simulink model "sampled_data_system"  (R2020a)
settings: Solver=VariableStepAuto  StartTime=0.0  StopTime=20  RelTol=1e-3
values from neighbouring files (symbols this model uses):
  B = 1 / k_m    (= 0.0517063081696)    [Teleop_parameters.m]    (also in base.mat; base_no_attrito.mat = 0; ci_siamo.mat; force_control.mat)
  Be = 5    [Teleop_parameters.m]    (also in base.mat = 0.5; base_no_attrito.mat = 0.5; ci_siamo.mat; force_control.mat = 0.5)
  Bh = 0.02    [Teleop_parameters.m]    (also in base.mat; base_no_attrito.mat; ci_siamo.mat; force_control.mat)
  D = 1    [Teleop_parameters.m]    (also in base.mat = 2; base_no_attrito.mat = 2; force_control.mat = 2; force_control_senza_attrito.mat = 2)
  Fc_h = 5    [Teleop_parameters.m]    (also in base.mat; base_no_attrito.mat; ci_siamo.mat; force_control.mat)
  J = tau_m / k_m    (= 0.0629265770424)    [Teleop_parameters.m]    (also in base.mat; base_no_attrito.mat; ci_siamo.mat; force_control.mat)
  J_r = J + J * 0.5    (= 0.0943898655636)    [Teleop_parameters.m]    (also in base.mat; base_no_attrito.mat; ci_siamo.mat = 0.0629265770424; force_control.mat)
  Jh = 0.02    [Teleop_parameters.m]    (also in base.mat; base_no_attrito.mat; ci_siamo.mat; force_control.mat)
  Kc2v_m = 2    [Teleop_parameters.m]    (also in base.mat; base_no_attrito.mat; ci_siamo.mat; force_control.mat)
  Kc2v_s = 2    [Teleop_parameters.m]    (also in base.mat; base_no_attrito.mat; ci_siamo.mat; force_control.mat)
  Kd_h = 1    [Teleop_parameters.m]    (also in base.mat; base_no_attrito.mat; ci_siamo.mat = 10; force_control.mat)
  Kd_m = 1    [Teleop_parameters.m]    (also in base.mat; base_no_attrito.mat; ci_siamo.mat = 0.005; force_control.mat)
  Kd_s = 1    [Teleop_parameters.m]    (also in base.mat; base_no_attrito.mat; ci_siamo.mat = 0.5; force_control.mat)
  Ke = 10    [Teleop_parameters.m]    (also in base.mat; base_no_attrito.mat; ci_siamo.mat; force_control.mat)
  Kp_h = 1.2    [Teleop_parameters.m]    (also in base.mat; base_no_attrito.mat; ci_siamo.mat = 10; force_control.mat)
  Kp_m = 1    [Teleop_parameters.m]    (also in base.mat; base_no_attrito.mat; ci_siamo.mat = 0.01; force_control.mat)
  Kp_s = 1    [Teleop_parameters.m]    (also in base.mat; base_no_attrito.mat; ci_siamo.mat; force_control.mat)
  Kt2c_m = 1.182    [Teleop_parameters.m]    (also in base.mat; base_no_attrito.mat; ci_siamo.mat; force_control.mat)
  Kt2c_s = 1.182    [Teleop_parameters.m]    (also in base.mat; base_no_attrito.mat; ci_siamo.mat; force_control.mat)
  Kv_fc = 0    [Teleop_parameters.m]    (also in base.mat; base_no_attrito.mat; ci_siamo.mat = 10; force_control.mat = 30)
  lArm_m = 0.1    [Teleop_parameters.m]    (also in base.mat; base_no_attrito.mat; ci_siamo.mat; force_control.mat)
  lArm_s = 0.1    [Teleop_parameters.m]    (also in base.mat; base_no_attrito.mat; ci_siamo.mat; force_control.mat)
  qe = 0.5    [Teleop_parameters.m]    (also in base.mat = 5; base_no_attrito.mat = 5; ci_siamo.mat; force_control.mat = 5)
  Ts = 0.002    [Teleop_parameters.m]    (also in base.mat; base_no_attrito.mat; ci_siamo.mat; force_control.mat)
undefined symbols (not defined in the file or in its folder): DiscIntNeverNeededParam
settings Model: Creator=gbagolin  LastModifiedBy=giova
settings SolverCC: AlgebraicLoopSolver=LineSearch

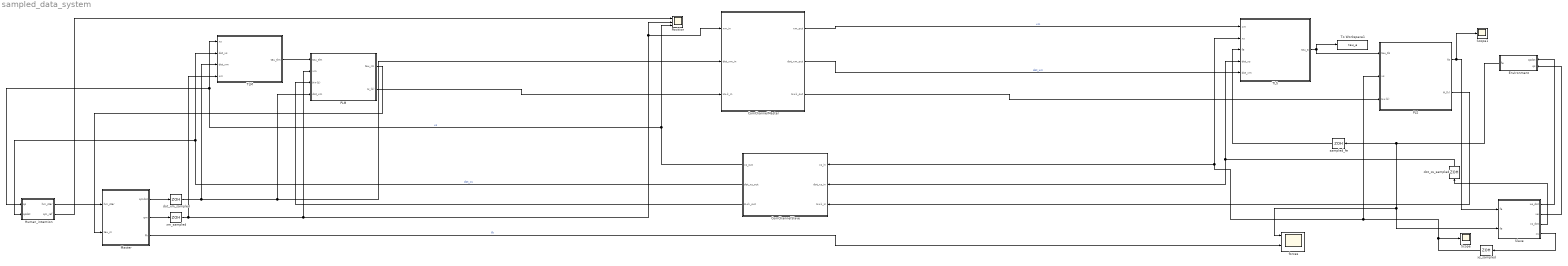
== system sampled_data_system ==
  ComChannelMaster : Subsystem
  ComChannelSlave : Subsystem
  Environment : Subsystem
  Human_intention : Subsystem
  Master : Subsystem
  PLM : Subsystem
  PLS : Subsystem
  Position : Scope  NumInputPorts=3
  Scope : Scope
  Scope1 : Scope
  Slave : Subsystem
  TLM : Subsystem
  TLS : Subsystem
  To Workspace1 : ToWorkspace  VariableName=tau_a  SaveFormat=Timeseries  SampleTime=-1
  dot_xm_sampled : ZeroOrderHold  SampleTime=Ts
  dot_xs_sampled : ZeroOrderHold  SampleTime=Ts
  forces : Scope  NumInputPorts=5
  sampled_fe : ZeroOrderHold  SampleTime=-1
  xm_sampled : ZeroOrderHold  SampleTime=Ts
  xs_sampled : ZeroOrderHold  SampleTime=Ts
  wires:
  Human_intention/1(hm_star) -> Master/1(hm_star)
  Environment/1(fe) -> Slave/2(fe), forces/1, sampled_fe/1
  Slave/3(xs_dot) -> dot_xs_sampled/1
  Slave/1(xe_dot) -> Environment/1(qsdot)
  Slave/2(xe) -> Environment/2(qs)
  Slave/4(xs) -> xs_sampled/1
  Master/2(qm) -> xm_sampled/1
  Human_intention/2(qm_ref) -> Position/1
  Master/3(fh) -> forces/4  "fh"
  xm_sampled/1 -> Position/2, ComChannelMaster/1(xm_in), PLM/2(xm), TLM/4(xm)
  xs_sampled/1 -> Scope/1, TLS/2(xs), ComChannelSlave/1(xs_in), PLS/2(xs)
  dot_xs_sampled/1 -> ComChannelSlave/2(dot_xs_in), TLS/4(dot_xs)
  TLS/1(tau_a) -> PLS/1(tau_tls), To Workspace1/1
  dot_xm_sampled/1 -> ComChannelMaster/2(dot_xm_in), PLM/4(dot_xm), TLM/3(dot_xm)
  sampled_fe/1 -> TLS/3(fe)
  Master/1(qmdot) -> dot_xm_sampled/1
  TLM/1(tau_tlm) -> PLM/1(tau_tlm)
  PLM/1(tau_rm) -> Master/2(tau_m)
  ComChannelMaster/1(xm_out) -> TLS/1(xm)  "xm"
  ComChannelMaster/2(dot_xm_out) -> TLS/5(dot_xm)  "dot_xm"
  ComChannelSlave/1(xs_out) -> TLM/1(xs), Human_intention/1(qs), Position/3  "xs"
  ComChannelSlave/2(dot_xs_out) -> Human_intention/2(qsdot), TLM/2(dot_xs)  "dot_xs"
  ComChannelSlave/3(H+k_out) -> PLM/3(H+(k))
  ComChannelMaster/3(H+k_out) -> PLS/3(H+(k))
  PLS/1(fa) -> Scope1/1, Slave/1(fa)
  PLM/2(H_(k)) -> ComChannelMaster/3(H+k_in)
  PLS/2(H_(k)) -> ComChannelSlave/3(H+k_in)

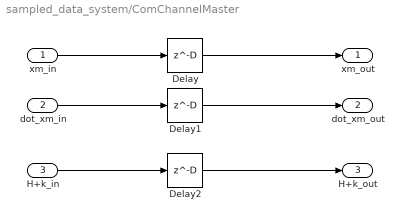
== system sampled_data_system/ComChannelMaster ==
  xm_in : Inport
  dot_xm_in : Inport  Port=2
  H+k_in : Inport  Port=3
  Delay : Delay  DelayLength=D  SampleTime=Ts
  Delay1 : Delay  DelayLength=D  SampleTime=Ts
  Delay2 : Delay  DelayLength=D  SampleTime=Ts
  xm_out : Outport
  dot_xm_out : Outport  Port=2
  H+k_out : Outport  Port=3
  wires:
  xm_in/1 -> Delay/1
  dot_xm_in/1 -> Delay1/1
  H+k_in/1 -> Delay2/1
  Delay/1 -> xm_out/1
  Delay1/1 -> dot_xm_out/1
  Delay2/1 -> H+k_out/1

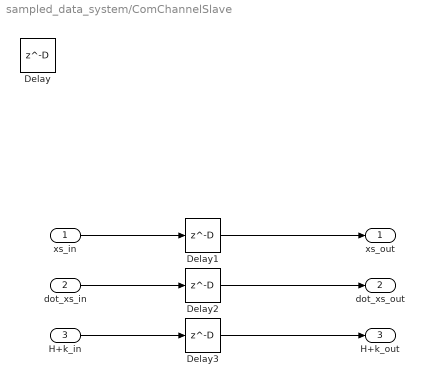
== system sampled_data_system/ComChannelSlave ==
  xs_in : Inport
  dot_xs_in : Inport  Port=2
  H+k_in : Inport  Port=3
  Delay{,1..3} (4 alike) : Delay  DelayLength=D  SampleTime=Ts
  xs_out : Outport
  dot_xs_out : Outport  Port=2
  H+k_out : Outport  Port=3
  wires:
  xs_in/1 -> Delay1/1
  dot_xs_in/1 -> Delay2/1
  H+k_in/1 -> Delay3/1
  Delay1/1 -> xs_out/1
  Delay2/1 -> dot_xs_out/1
  Delay3/1 -> H+k_out/1

== system sampled_data_system/Environment ==
  note: force
  qsdot : Inport
  qs : Inport  Port=2
  To Workspace : ToWorkspace  VariableName=fe  SaveFormat=Timeseries  SampleTime=-1
  c1 : Constant  Value=Be  SampleTime=0
  c2 : Constant  Value=Ke  SampleTime=0
  env : MATLAB Function  TreatAsAtomicUnit=on
  qe : Constant  Value=qe  SampleTime=0
  fe : Outport  VectorParamsAs1DForOutWhenUnconnected=off
  wires:
  qe/1 -> env/3(qe)
  c1/1 -> env/2(Be)
  c2/1 -> env/1(Ke)
  qs/1 -> env/4(qs)
  qsdot/1 -> env/5(qsdot)
  env/1(fE) -> To Workspace/1, fe/1

== system sampled_data_system/Human_intention ==
  qs : Inport
  qsdot : Inport  Port=2
  Operator (intention) : Subsystem
  Subsystem : Subsystem
  To Workspace : ToWorkspace  VariableName=qm_ref  SaveFormat=Timeseries  SampleTime=-1
  To Workspace1 : ToWorkspace  VariableName=fh  SaveFormat=Timeseries  SampleTime=-1
  hm_star : Outport
  qm_ref : Outport  Port=2
  wires:
  Subsystem/1(qm_ref) -> To Workspace/1, Operator (intention)/3(qm_ref), qm_ref/1
  Subsystem/2(qmdot_ref) -> Operator (intention)/4(qmdot_ref)
  Operator (intention)/1(hm_star) -> To Workspace1/1, hm_star/1
  qs/1 -> Operator (intention)/1(qs)
  qsdot/1 -> Operator (intention)/2(qsdot)

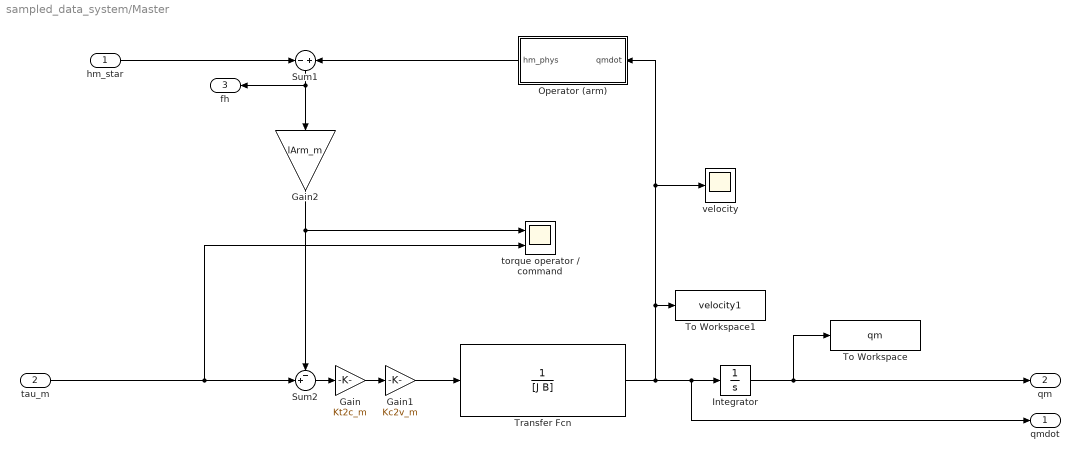
== system sampled_data_system/Master ==
  hm_star : Inport
  tau_m : Inport  Port=2
  Gain : Gain  Gain=Kt2c_m
  Gain1 : Gain  Gain=Kc2v_m
  Gain2 : Gain  Gain=lArm_m
  Integrator : Integrator
  Operator (arm) : Subsystem
  Sum1 : Sum  Inputs=-+
  Sum2 : Sum  Inputs=-+|
  To Workspace : ToWorkspace  VariableName=qm  SaveFormat=Timeseries  SampleTime=-1
  To Workspace1 : ToWorkspace  VariableName=velocity1  SaveFormat=Timeseries  SampleTime=-1
  Transfer Fcn : TransferFcn  Denominator=[J B]
  torque operator / command : Scope  NumInputPorts=2
  velocity : Scope
  qmdot : Outport
  qm : Outport  Port=2
  fh : Outport  Port=3
  wires:
  Integrator/1 -> To Workspace/1, qm/1
  Operator (arm)/1(hm_phys) -> Sum1/2
  Sum1/1 -> Gain2/1, fh/1
  Transfer Fcn/1 -> Operator (arm)/1(qmdot), velocity/1, To Workspace1/1, qmdot/1, Integrator/1
  hm_star/1 -> Sum1/1
  Sum2/1 -> Gain/1
  Gain/1 -> Gain1/1
  Gain1/1 -> Transfer Fcn/1
  Gain2/1 -> Sum2/1, torque operator / command/1
  tau_m/1 -> Sum2/2, torque operator / command/2

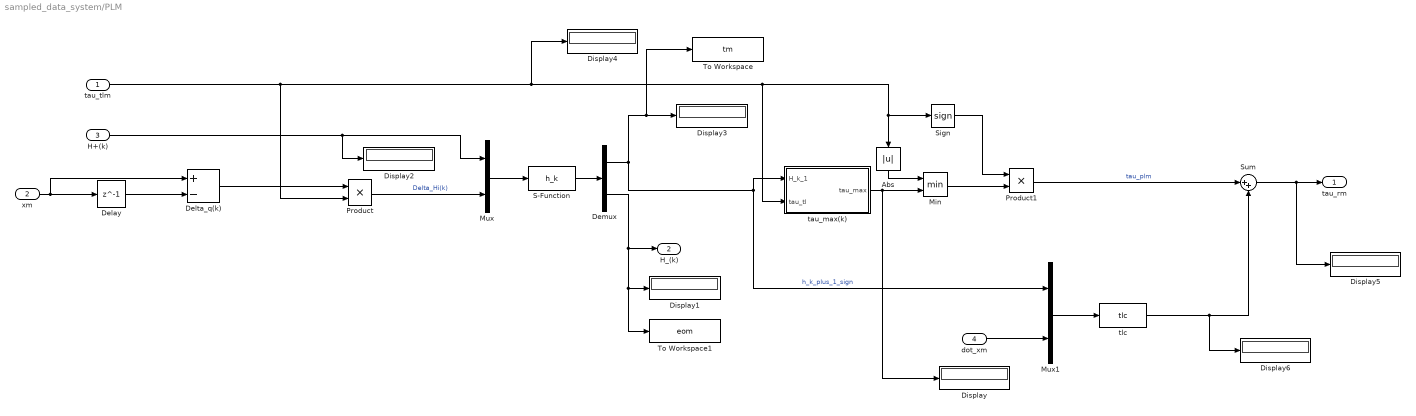
== system sampled_data_system/PLM ==
  tau_tlm : Inport
  xm : Inport  Port=2
  H+(k) : Inport  Port=3
  dot_xm : Inport  Port=4
  Abs : Abs
  Delay : Delay  DelayLength=1  SampleTime=Ts
  Delta_q(k) : Sum  Inputs=+-
  Demux : Demux  Outputs=2
  Display{,1..6} (7 alike) : Display
  Min : MinMax  Inputs=2
  Mux : Mux  Inputs=2
  Mux1 : Mux  Inputs=2
  Product : Product
  Product1 : Product
  S-Function : S-Function  FunctionName=h_k  Parameters=param  SFunctionDeploymentMode=off  EnableBusSupport=off
  Sign : Signum
  Sum : Sum  Inputs=|++
  To Workspace : ToWorkspace  VariableName=tm  SaveFormat=Timeseries  SampleTime=-1
  To Workspace1 : ToWorkspace  VariableName=eom  SaveFormat=Timeseries  SampleTime=-1
  tau_max(k) : MATLAB Function  TreatAsAtomicUnit=on
  tlc : S-Function  FunctionName=tlc  Parameters=param  SFunctionDeploymentMode=off  EnableBusSupport=off
  tau_rm : Outport
  H_(k) : Outport  Port=2
  wires:
  Delta_q(k)/1 -> Product/1
  xm/1 -> Delay/1, Delta_q(k)/1
  Product/1 -> Mux/2  "Delta_Hi(k)"
  H+(k)/1 -> Mux/1, Display2/1
  tau_max(k)/1(tau_max) -> Display/1, Min/2
  Min/1 -> Product1/2
  Sign/1 -> Product1/1
  Product1/1 -> Sum/1  "tau_plm"
  dot_xm/1 -> Mux1/2
  tlc/1 -> Display6/1, Sum/2
  Mux/1 -> S-Function/1
  Delay/1 -> Delta_q(k)/2
  S-Function/1 -> Demux/1
  Demux/1 -> Mux1/1, tau_max(k)/1(H_k_1), To Workspace/1, Display3/1  "h_k_plus_1_sign"
  Demux/2 -> Display1/1, To Workspace1/1, H_(k)/1
  Mux1/1 -> tlc/1
  tau_tlm/1 -> Product/2, tau_max(k)/2(tau_tl), Sign/1, Abs/1, Display4/1
  Abs/1 -> Min/1
  Sum/1 -> Display5/1, tau_rm/1

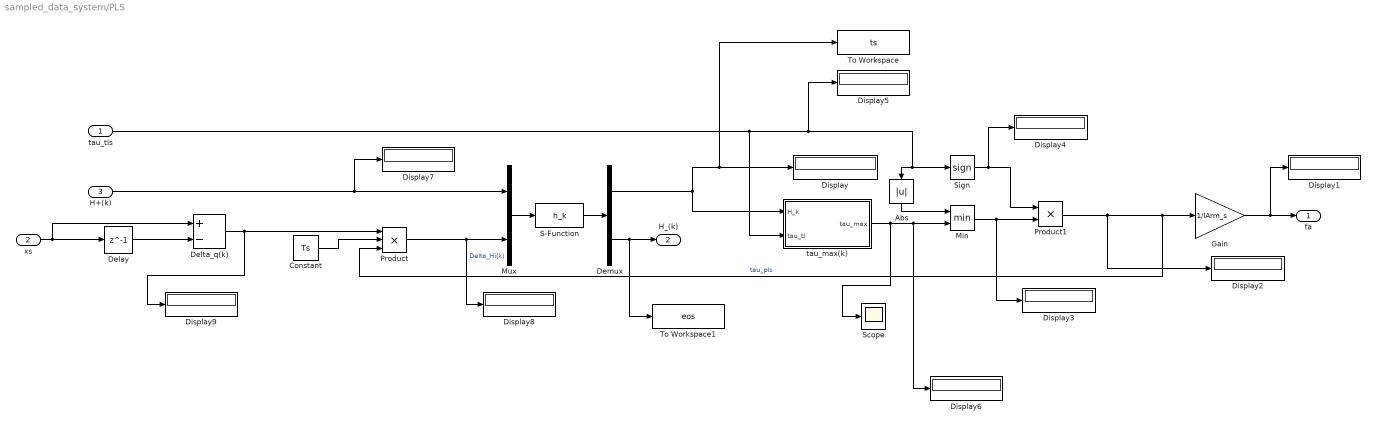
== system sampled_data_system/PLS ==
  tau_tls : Inport
  xs : Inport  Port=2
  H+(k) : Inport  Port=3
  Abs : Abs
  Constant : Constant  Value=Ts
  Delay : Delay  DelayLength=1  SampleTime=Ts
  Delta_q(k) : Sum  Inputs=+-
  Demux : Demux  Outputs=2
  Display{,1..9} (10 alike) : Display
  Gain : Gain  Gain=1/lArm_s
  Min : MinMax  Inputs=2
  Mux : Mux  Inputs=2
  Product : Product  Inputs=3
  Product1 : Product
  S-Function : S-Function  FunctionName=h_k  Parameters=param  SFunctionDeploymentMode=off  EnableBusSupport=off
  Scope : Scope
  Sign : Signum
  To Workspace : ToWorkspace  VariableName=ts  SaveFormat=Timeseries  SampleTime=-1
  To Workspace1 : ToWorkspace  VariableName=eos  SaveFormat=Timeseries  SampleTime=-1
  tau_max(k) : MATLAB Function  TreatAsAtomicUnit=on
  fa : Outport
  H_(k) : Outport  Port=2
  wires:
  Product1/1 -> Display2/1, Product/3, Gain/1  "tau_pls"
  Sign/1 -> Display4/1, Product1/1
  tau_max(k)/1(tau_max) -> Scope/1, Display6/1, Min/2
  xs/1 -> Delay/1, Delta_q(k)/1
  Min/1 -> Display3/1, Product1/2
  Delta_q(k)/1 -> Display9/1, Product/1
  Gain/1 -> Display1/1, fa/1
  Mux/1 -> S-Function/1
  Product/1 -> Display8/1, Mux/2  "Delta_Hi(k)"
  H+(k)/1 -> Display7/1, Mux/1
  S-Function/1 -> Demux/1
  Demux/1 -> To Workspace/1, Display/1, tau_max(k)/1(H_k)
  Demux/2 -> To Workspace1/1, H_(k)/1
  Delay/1 -> Delta_q(k)/2
  tau_tls/1 -> tau_max(k)/2(tau_tl), Abs/1, Sign/1, Display5/1
  Abs/1 -> Min/1
  Constant/1 -> Product/2

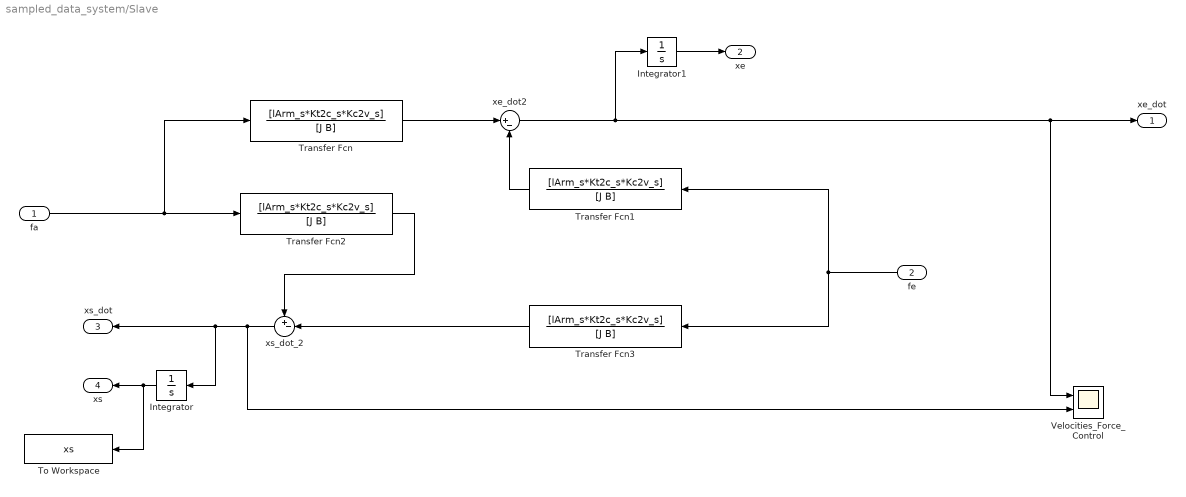
== system sampled_data_system/Slave ==
  fa : Inport
  fe : Inport  Port=2
  Integrator : Integrator
  Integrator1 : Integrator
  To Workspace : ToWorkspace  VariableName=xs  SaveFormat=Timeseries  SampleTime=-1
  Transfer Fcn{,1..3} (4 alike) : TransferFcn  Numerator=[lArm_s*Kt2c_s*Kc2v_s]  Denominator=[J B]
  Velocities_Force_Control : Scope  NumInputPorts=2
  xe_dot2 : Sum  Inputs=|+-
  xs_dot_2 : Sum  Inputs=+-|
  xe_dot : Outport
  xe : Outport  Port=2
  xs_dot : Outport  Port=3
  xs : Outport  Port=4
  wires:
  fa/1 -> Transfer Fcn2/1, Transfer Fcn/1
  Transfer Fcn/1 -> xe_dot2/1
  xe_dot2/1 -> Integrator1/1, xe_dot/1, Velocities_Force_Control/1
  Transfer Fcn1/1 -> xe_dot2/2
  Transfer Fcn3/1 -> xs_dot_2/2
  Transfer Fcn2/1 -> xs_dot_2/1
  xs_dot_2/1 -> Velocities_Force_Control/2, Integrator/1, xs_dot/1
  fe/1 -> Transfer Fcn1/1, Transfer Fcn3/1
  Integrator/1 -> To Workspace/1, xs/1
  Integrator1/1 -> xe/1

== system sampled_data_system/TLM ==
  xs : Inport
  dot_xs : Inport  Port=2
  dot_xm : Inport  Port=3
  xm : Inport  Port=4
  PD controller : Subsystem
  tau_tlm : Outport
  wires:
  PD controller/1(tau_c) -> tau_tlm/1
  dot_xm/1 -> PD controller/2(dot_x)
  dot_xs/1 -> PD controller/4(dot_xd)
  xs/1 -> PD controller/3(xd)
  xm/1 -> PD controller/1(x)

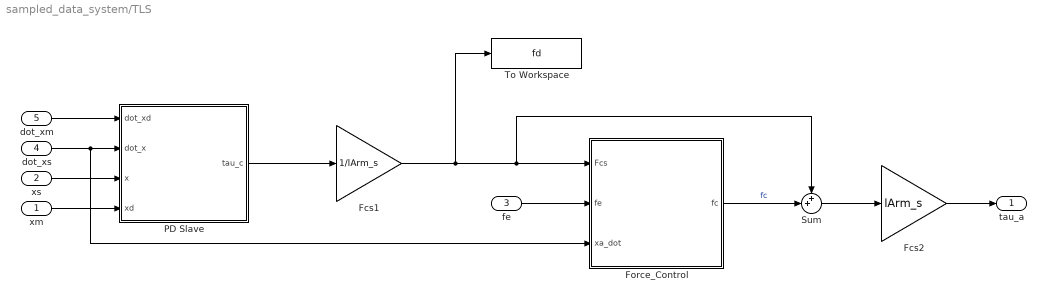
== system sampled_data_system/TLS ==
  xm : Inport
  xs : Inport  Port=2
  fe : Inport  Port=3
  dot_xs : Inport  Port=4
  dot_xm : Inport  Port=5
  Fcs1 : Gain  Gain=1/lArm_s
  Fcs2 : Gain  Gain=lArm_s
  Force_Control : Subsystem
  PD Slave : Subsystem
  Sum : Sum  Inputs=++|
  To Workspace : ToWorkspace  VariableName=fd  SaveFormat=Timeseries  SampleTime=-1
  tau_a : Outport
  wires:
  xs/1 -> PD Slave/3(x)
  Fcs1/1 -> To Workspace/1, Sum/1, Force_Control/1(Fcs)
  dot_xm/1 -> PD Slave/1(dot_xd)
  fe/1 -> Force_Control/2(fe)
  xm/1 -> PD Slave/4(xd)
  dot_xs/1 -> Force_Control/3(xa_dot), PD Slave/2(dot_x)
  PD Slave/1(tau_c) -> Fcs1/1
  Force_Control/1(fc) -> Sum/2  "fc"
  Sum/1 -> Fcs2/1
  Fcs2/1 -> tau_a/1

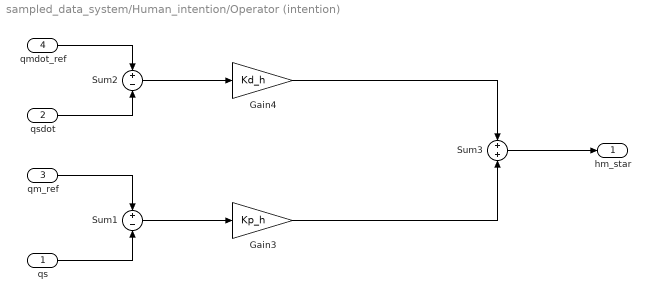
== system sampled_data_system/Human_intention/Operator (intention) ==
  qs : Inport
  qsdot : Inport  Port=2
  qm_ref : Inport  Port=3
  qmdot_ref : Inport  Port=4
  Gain3 : Gain  Gain=Kp_h
  Gain4 : Gain  Gain=Kd_h
  Sum1 : Sum  Inputs=+|-
  Sum2 : Sum  Inputs=+|-
  Sum3 : Sum  Inputs=+|+
  hm_star : Outport  VectorParamsAs1DForOutWhenUnconnected=off
  wires:
  qs/1 -> Sum1/2
  qm_ref/1 -> Sum1/1
  qmdot_ref/1 -> Sum2/1
  Sum1/1 -> Gain3/1
  qsdot/1 -> Sum2/2
  Sum2/1 -> Gain4/1
  Gain4/1 -> Sum3/1
  Gain3/1 -> Sum3/2
  Sum3/1 -> hm_star/1

== system sampled_data_system/Human_intention/Subsystem ==
  Derivative1 : Derivative  CoefficientInTFapproximation=0.001
  Manual Switch : ManualSwitch  CurrentSetting=0
  Sine Wave : Sin  SampleTime=0
  Step : Step  SampleTime=0
  low-pass filter : TransferFcn  Numerator=[2*pi*Fc_h]  Denominator=[1 2*pi*Fc_h]
  qm_ref : Outport
  qmdot_ref : Outport  Port=2
  wires:
  low-pass filter/1 -> Manual Switch/2
  Manual Switch/1 -> qm_ref/1, Derivative1/1
  Derivative1/1 -> qmdot_ref/1  "qmdot_ref"
  Step/1 -> low-pass filter/1
  Sine Wave/1 -> Manual Switch/1

== system sampled_data_system/Master/Operator (arm) ==
  note: force
  qmdot : Inport
  Derivative : Derivative  CoefficientInTFapproximation=0.001
  Gain1 : Gain  Gain=Jh
  Gain2 : Gain  Gain=Bh
  Sum : Sum  Inputs=+|+
  hm_phys : Outport  VectorParamsAs1DForOutWhenUnconnected=off
  wires:
  qmdot/1 -> Gain2/1, Derivative/1
  Sum/1 -> hm_phys/1
  Derivative/1 -> Gain1/1
  Gain2/1 -> Sum/1
  Gain1/1 -> Sum/2

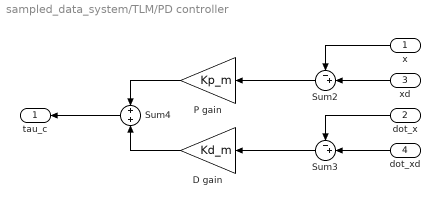
== system sampled_data_system/TLM/PD controller ==
  x : Inport
  dot_x : Inport  Port=2
  xd : Inport  Port=3
  dot_xd : Inport  Port=4
  D gain : Gain  Gain=Kd_m
  P gain : Gain  Gain=Kp_m
  Sum2 : Sum  Inputs=-+|
  Sum3 : Sum  Inputs=-+|
  Sum4 : Sum
  tau_c : Outport  VectorParamsAs1DForOutWhenUnconnected=off
  wires:
  D gain/1 -> Sum4/2
  dot_x/1 -> Sum3/1
  dot_xd/1 -> Sum3/2
  x/1 -> Sum2/1
  xd/1 -> Sum2/2
  Sum3/1 -> D gain/1
  P gain/1 -> Sum4/1
  Sum4/1 -> tau_c/1
  Sum2/1 -> P gain/1

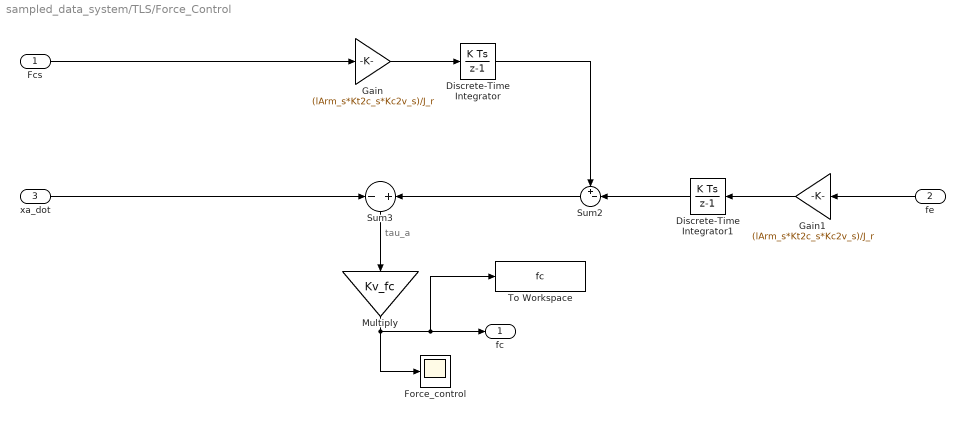
== system sampled_data_system/TLS/Force_Control ==
  note: tau_a
  Fcs : Inport
  fe : Inport  Port=2
  xa_dot : Inport  Port=3
  Discrete-Time Integrator : DiscreteIntegrator  SampleTime=Ts  ICPrevOutput=DiscIntNeverNeededParam  ICPrevScaledInput=DiscIntNeverNeededParam
  Discrete-Time Integrator1 : DiscreteIntegrator  SampleTime=Ts  ICPrevOutput=DiscIntNeverNeededParam  ICPrevScaledInput=DiscIntNeverNeededParam
  Force_control : Scope
  Gain : Gain  Gain=(lArm_s*Kt2c_s*Kc2v_s)/J_r
  Gain1 : Gain  Gain=(lArm_s*Kt2c_s*Kc2v_s)/J_r
  Multiply : Gain  Gain=Kv_fc
  Sum2 : Sum  Inputs=+-|
  Sum3 : Sum  Inputs=-|+
  To Workspace : ToWorkspace  VariableName=fc  SaveFormat=Timeseries  SampleTime=-1
  fc : Outport
  wires:
  Discrete-Time Integrator1/1 -> Sum2/2
  Sum2/1 -> Sum3/2
  Sum3/1 -> Multiply/1
  Multiply/1 -> To Workspace/1, fc/1, Force_control/1
  Fcs/1 -> Gain/1
  fe/1 -> Gain1/1
  xa_dot/1 -> Sum3/1
  Discrete-Time Integrator/1 -> Sum2/1
  Gain/1 -> Discrete-Time Integrator/1
  Gain1/1 -> Discrete-Time Integrator1/1

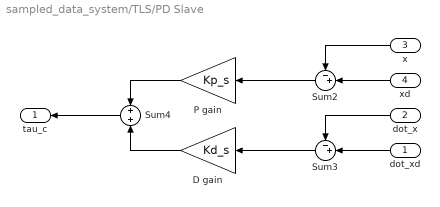
== system sampled_data_system/TLS/PD Slave ==
  dot_xd : Inport
  dot_x : Inport  Port=2
  x : Inport  Port=3
  xd : Inport  Port=4
  D gain : Gain  Gain=Kd_s
  P gain : Gain  Gain=Kp_s
  Sum2 : Sum  Inputs=-+|
  Sum3 : Sum  Inputs=-+|
  Sum4 : Sum
  tau_c : Outport  VectorParamsAs1DForOutWhenUnconnected=off
  wires:
  D gain/1 -> Sum4/2
  dot_x/1 -> Sum3/1
  dot_xd/1 -> Sum3/2
  x/1 -> Sum2/1
  xd/1 -> Sum2/2
  Sum3/1 -> D gain/1
  P gain/1 -> Sum4/1
  Sum4/1 -> tau_c/1
  Sum2/1 -> P gain/1

== matlab function sampled_data_system/PLM/tau_max(k) ==
  data: H_k_1 input; tau_max output; tau_tl input
function tau_max = fcn(H_k_1,tau_tl)
    if H_k_1 <= 0
        tau_max = 0; 
    else
        tau_max = tau_tl;
    end

== matlab function sampled_data_system/PLS/tau_max(k) ==
  data: H_k input; tau_max output; tau_tl input
function tau_max = fcn(H_k,tau_tl)
    if H_k <= 0
        tau_max = 0; 
    else
        tau_max = tau_tl;
    end

== matlab function sampled_data_system/Environment/env ==
  data: Ke input; Be input; qe input; qs input; fE output; qsdot input
function fE  = environment(Ke, Be, qe, qs, qsdot)
if qs > qe
   fE = Ke * (qs - qe) + Be * qsdot;
else
   fE = 0;
end
